simulink model "EMPlanner_cs_old"  (R2023a)
settings: Solver=ode5  StartTime=0.0  StopTime=60  FixedStep=1/1000  RelTol=1e-3
PreLoadFcn:
  | mbxruntime.callbacks.PreLoadFcn(bdroot);
PostLoadFcn:
  | mbxruntime.callbacks.PostLoadFcn(bdroot);
InitFcn:
  | mbxruntime.callbacks.InitFcn(bdroot);
StartFcn:
  | mbxruntime.callbacks.StartFcn(bdroot);
StopFcn:
  | mbxruntime.callbacks.StopFcn(bdroot);
model workspace: external: MAT-File .\EMPlanner_cs_hws.mat (data not in the file)
values from neighbouring files (symbols this model uses):
  c_factor = 43.75    [emplanner_init.m]
  cf = -64276.3    [emplanner_init.m]
  cr = -64276.3    [emplanner_init.m]
  KD_PID_distance = 0.0    (= 0)    [emplanner_init.m]
  KD_PID_speed = 0    [emplanner_init.m]
  KI_PID_distance = 0.0    (= 0)    [emplanner_init.m]
  KI_PID_speed = 0    [emplanner_init.m]
  KP_PID_distance = 0.5    [emplanner_init.m]
  KP_PID_speed = 1.8    [emplanner_init.m]
  la = 0.5989    [emplanner_init.m]
  lb = 1.1979-0.5989    (= 0.599)    [emplanner_init.m]
  LQR_K1 = k(:,1)'    [emplanner_init.m]
  LQR_K2 = k(:,2)'    [emplanner_init.m]
  LQR_K3 = k(:,3)'    [emplanner_init.m]
  LQR_K4 = k(:,4)'    [emplanner_init.m]
  m = 375.8    [emplanner_init.m]
  vx_break_point = zeros(1,5000)    [emplanner_init.m]
undefined symbols (not defined in the file or in its folder): aubr, DiscIntNeverNeededParam, EMPlanner_cs_27357ced727cddc2, EMPlanner_cs_3a309230b46bf2dd, EMPlanner_cs_4725e6271df7126f, EMPlanner_cs_7cd0898d5750b5ce, EMPlanner_cs_9531ed1ae61b92f2, EMPlanner_cs_Box_10_Dynamics_Empty_STATE_Box_10_Pitch0, EMPlanner_cs_Box_10_Dynamics_Empty_STATE_Box_10_Roll0, EMPlanner_cs_Box_10_Dynamics_Empty_STATE_Box_10_x0, EMPlanner_cs_Box_10_Dynamics_Empty_STATE_Box_10_y0, EMPlanner_cs_Box_10_Dynamics_Empty_STATE_Box_10_Yaw0, EMPlanner_cs_Box_10_Dynamics_Empty_STATE_Box_10_z0, EMPlanner_cs_Box_1_Path_pathUniqueID, EMPlanner_cs_Box_1_SpeedProfile_speedProfileUniqueID, EMPlanner_cs_Box_2_Path_pathUniqueID, EMPlanner_cs_Box_2_SpeedProfile_speedProfileUniqueID, EMPlanner_cs_Box_3_Path_pathUniqueID, EMPlanner_cs_Box_3_SpeedProfile_speedProfileUniqueID, EMPlanner_cs_Box_4_Path_pathUniqueID, EMPlanner_cs_Box_4_SpeedProfile_speedProfileUniqueID, EMPlanner_cs_Box_5_Dynamics_Empty_STATE_Box_5_Pitch0, EMPlanner_cs_Box_5_Dynamics_Empty_STATE_Box_5_Roll0, EMPlanner_cs_Box_5_Dynamics_Empty_STATE_Box_5_x0, EMPlanner_cs_Box_5_Dynamics_Empty_STATE_Box_5_y0, EMPlanner_cs_Box_5_Dynamics_Empty_STATE_Box_5_Yaw0, EMPlanner_cs_Box_5_Dynamics_Empty_STATE_Box_5_z0, EMPlanner_cs_Box_6_Path_pathUniqueID, EMPlanner_cs_Box_6_SpeedProfile_speedProfileUniqueID, EMPlanner_cs_Box_7_Dynamics_Empty_STATE_Box_7_Pitch0, EMPlanner_cs_Box_7_Dynamics_Empty_STATE_Box_7_Roll0, EMPlanner_cs_Box_7_Dynamics_Empty_STATE_Box_7_x0, EMPlanner_cs_Box_7_Dynamics_Empty_STATE_Box_7_y0, EMPlanner_cs_Box_7_Dynamics_Empty_STATE_Box_7_Yaw0, EMPlanner_cs_Box_7_Dynamics_Empty_STATE_Box_7_z0, EMPlanner_cs_Box_8_Dynamics_Empty_STATE_Box_8_Pitch0, EMPlanner_cs_Box_8_Dynamics_Empty_STATE_Box_8_Roll0, EMPlanner_cs_Box_8_Dynamics_Empty_STATE_Box_8_x0, EMPlanner_cs_Box_8_Dynamics_Empty_STATE_Box_8_y0, EMPlanner_cs_Box_8_Dynamics_Empty_STATE_Box_8_Yaw0, EMPlanner_cs_Box_8_Dynamics_Empty_STATE_Box_8_z0, EMPlanner_cs_Box_9_Dynamics_Empty_STATE_Box_9_Pitch0, EMPlanner_cs_Box_9_Dynamics_Empty_STATE_Box_9_Roll0, EMPlanner_cs_Box_9_Dynamics_Empty_STATE_Box_9_x0, EMPlanner_cs_Box_9_Dynamics_Empty_STATE_Box_9_y0, EMPlanner_cs_Box_9_Dynamics_Empty_STATE_Box_9_Yaw0, EMPlanner_cs_Box_9_Dynamics_Empty_STATE_Box_9_z0, EMPlanner_cs_dca7ae789a013f83, global_path_x, global_path_y, mbxruntime, rack_displacement, right_wheel_ground, tablebr, vubr
libraries: PreScanSimulinkLibrary x12, Solver_SF x1
(part 5 of 9)

== system EMPlanner_cs_old/modular_bus_1/Dynamics_UserSpecified/MuxState ==
  note: mode: Dynamics
  note: mode: Positioning
  note: mode: Dynamics
      | VelVEHICLE
      | wrt VEH
  note: AnglesVEHICLE
      | wrtGLOB
  note: For state mode 'Dynamic' positions
      | are not taken into account, as they
      | are computed by integrating velocity.
      | Click annotation for Help.
  x [m] : Inport  SampleTime=TimeStep
  y [m] : Inport  Port=2  SampleTime=TimeStep
  z [m] : Inport  Port=3  SampleTime=TimeStep
  dx [m/s] : Inport  Port=4  SampleTime=TimeStep
  dy [m/s] : Inport  Port=5  SampleTime=TimeStep
  dz [m/s] : Inport  Port=6  SampleTime=TimeStep
  R [rad] : Inport  Port=7  SampleTime=TimeStep
  P [rad] : Inport  Port=8  SampleTime=TimeStep
  Y [rad] : Inport  Port=9  SampleTime=TimeStep
  Constant : Constant  DisableCoverage=on  Value=positioningmode
  Discrete-Time Integrator : DiscreteIntegrator  SampleTime=TimeStep  ICPrevOutput=DiscIntNeverNeededParam  ICPrevScaledInput=DiscIntNeverNeededParam
  Ground : Ground
  Ground1 : Ground
  Mux1 : Mux  Inputs=[3 3]
  Mux2 : Mux  Inputs=3
  Mux3 : Mux  Inputs=3
  Mux4 : Mux  Inputs=3
  Mux5 : Mux  Inputs=[3 3]
  Mux6 : Mux  Inputs=[6 3]
  Switch : Switch  Threshold=0.5  SaturateOnIntegerOverflow=off  InputSameDT=off
  Transformation_BODY2GLOBAL : PreScanSimulinkLibrary/Simple_Vehicle_Dynamics/Chassis/MuxDynState/Transformation_BODY2GLOBAL  SystemSampleTime=-1  VariantActivationTime=update diagram  Latency=0  AutoFrameSizeCalculation=off
  mux3 : Mux  Inputs=3
  state : Outport
  wires:
  Constant/1 -> Switch/2
  Mux6/1 -> state/1
  Mux4/1 -> Mux1/1
  Mux5/1 -> Switch/3
  Mux1/1 -> Switch/1
  Switch/1 -> Mux6/1  "PosVeh wrt  GLOB"
  P [rad]/1 -> Mux3/2
  R [rad]/1 -> Mux3/1
  dz [m/s]/1 -> Mux2/3
  dy [m/s]/1 -> Mux2/2
  dx [m/s]/1 -> Mux2/1
  z [m]/1 -> Mux4/3
  y [m]/1 -> Mux4/2
  x [m]/1 -> Mux4/1
  Ground1/1 -> mux3/2  "pitch"
  Y [rad]/1 -> mux3/3, Mux3/3  "yaw"
  Mux3/1 -> Mux6/2
  Transformation_BODY2GLOBAL/1 -> Discrete-Time Integrator/1, Mux5/2  "VelVEH wrt  GLOB"
  mux3/1 -> Transformation_BODY2GLOBAL/2
  Ground/1 -> mux3/1  "roll"
  Mux2/1 -> Mux1/2, Transformation_BODY2GLOBAL/1
  Discrete-Time Integrator/1 -> Mux5/1  "PosVEH wrt  GLOB"

== system EMPlanner_cs_old/modular_bus_1/Dynamics_UserSpecified/STATE_modular_bus_1 ==
  State : Inport  SampleTime=TimeStep
  Bus Creator : BusCreator  Inputs=15  OutDataTypeStr=Bus: PRESCAN_STATEACTUATORDATA  NonVirtualBus=on
  Constant : Constant  Value=0
  Demux : Demux  Outputs=15
  Mux : Mux  Inputs=3
  Mux1 : Mux  Inputs=3
  Mux2 : Mux  Inputs=3
  iniBODYAngles wrtVEH [rad] : Constant  Value=Roll0  SampleTime=TimeStep
  iniBODYAngles wrtVEH [rad]1 : Constant  Value=Pitch0  SampleTime=TimeStep
  iniVEHAngles wrtGLOB [rad] : Constant  Value=Yaw0  SampleTime=TimeStep
  iniVEHposition wrtGLOB [m] : Constant  Value=x0  SampleTime=TimeStep
  iniVEHposition wrtGLOB [m]1 : Constant  Value=y0  SampleTime=TimeStep
  iniVEHposition wrtGLOB [m]2 : Constant  Value=z0  SampleTime=TimeStep
  state2FullState : PreScanSimulinkLibrary/state2FullState  SystemSampleTime=-1  VariantActivationTime=update diagram  Latency=0  AutoFrameSizeCalculation=off
  StateBus : Outport  OutDataTypeStr=Bus: PRESCAN_STATEACTUATORDATA
  wires:
  Mux2/1 -> state2FullState/4
  iniVEHAngles wrtGLOB [rad]/1 -> Mux2/3
  Mux1/1 -> state2FullState/3
  Constant/1 -> Mux2/1, Mux2/2, Mux1/3
  iniBODYAngles wrtVEH [rad]1/1 -> Mux1/2
  iniBODYAngles wrtVEH [rad]/1 -> Mux1/1
  Mux/1 -> state2FullState/2
  iniVEHposition wrtGLOB [m]2/1 -> Mux/3
  iniVEHposition wrtGLOB [m]/1 -> Mux/1
  iniVEHposition wrtGLOB [m]1/1 -> Mux/2
  Demux/15 -> Bus Creator/15  "AngularVelocityYaw"
  Demux/14 -> Bus Creator/14  "AngularVelocityPitch"
  Demux/13 -> Bus Creator/13  "AngularVelocityRoll"
  Demux/12 -> Bus Creator/12  "OrientationYaw"
  Demux/11 -> Bus Creator/11  "OrientationPitch"
  Demux/10 -> Bus Creator/10  "OrientationRoll"
  Demux/9 -> Bus Creator/9  "AccelerationZ"
  Demux/8 -> Bus Creator/8  "AccelerationY"
  Demux/7 -> Bus Creator/7  "AccelerationX"
  Demux/6 -> Bus Creator/6  "VelocityZ"
  Demux/5 -> Bus Creator/5  "VelocityY"
  Demux/4 -> Bus Creator/4  "VelocityX"
  Demux/3 -> Bus Creator/3  "PositionZ"
  Demux/2 -> Bus Creator/2  "PositionY"
  Demux/1 -> Bus Creator/1  "PositionX"
  state2FullState/1 -> Demux/1
  State/1 -> state2FullState/1
  Bus Creator/1 -> StateBus/1

== system EMPlanner_cs_old/modular_bus_1/SELF_Demux/compas converter ==
  rotz [rad] : Inport
  cart2compas : Subsystem
  rad2deg : Gain  Gain=180/pi
  heading [deg] : Outport
  wires:
  rad2deg/1 -> cart2compas/1(Angle [deg])
  rotz [rad]/1 -> rad2deg/1
  cart2compas/1(heading [deg]) -> heading [deg]/1

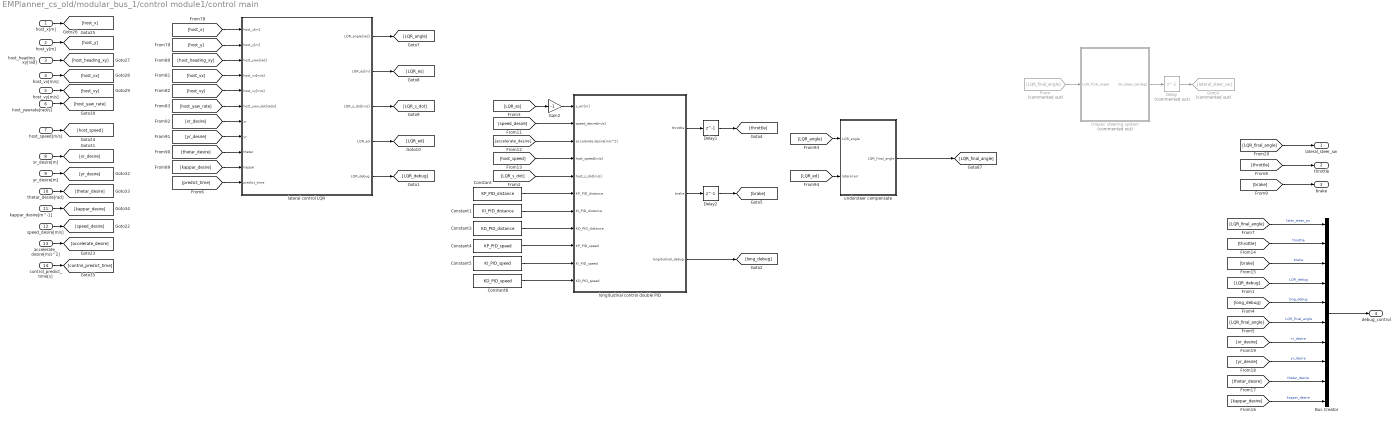
== system EMPlanner_cs_old/modular_bus_1/control module1/control main ==
  host_x[m] : Inport
  host_y[m] : Inport  Port=2
  host_heading_xy[rad] : Inport  Port=3
  host_vx[m/s] : Inport  Port=4
  host_vy[m/s] : Inport  Port=5
  host_yawrate[rad/s] : Inport  Port=6
  host_speed[m/s] : Inport  Port=7
  xr_desire[m] : Inport  Port=8
  yr_desire[m] : Inport  Port=9
  thetar_desire[rad] : Inport  Port=10
  kappar_desire[m^-1] : Inport  Port=11
  speed_desire[m/s] : Inport  Port=12
  accelerate_desire[m/s^2] : Inport  Port=13
  control_predict_time[s] : Inport  Port=14
  Bus Creator : BusCreator  Inputs=10
  Constant : Constant  Value=KP_PID_distance
  Constant1 : Constant  Value=KI_PID_distance
  Constant3 : Constant  Value=KD_PID_distance
  Constant4 : Constant  Value=KP_PID_speed
  Constant5 : Constant  Value=KI_PID_speed
  Constant6 : Constant  Value=KD_PID_speed
  Delay : Delay  Commented=on  DelayLength=1
  Delay1 : Delay  DelayLength=1
  Delay2 : Delay  DelayLength=1
  From : From  Commented=on  GotoTag=LQR_final_angle
  Gain2 : Gain  Gain=-1
  Goto3 : Goto  Commented=on  GotoTag=lateral_steer_sw
  chassic steering system : Subsystem  Commented=on
  lateral control LQR : Subsystem
  longitudinal control double PID : Subsystem
  understeer compensate : Subsystem
  lateral_steer_sw : Outport
  throttle : Outport  Port=2
  brake : Outport  Port=3
  debug_control : Outport  Port=4
  wires:
  [kappar_desire] -> Bus Creator/10  "kappar_desire"
  [thetar_desire] -> Bus Creator/9  "thetar_desire"
  [yr_desire] -> Bus Creator/8  "yr_desire"
  [xr_desire] -> Bus Creator/7  "xr_desire"
  Bus Creator/1 -> debug_control/1
  [LQR_final_angle] -> Bus Creator/6  "LQR_final_angle"
  [long_debug] -> Bus Creator/5  "long_debug"
  [LQR_debug] -> Bus Creator/4  "LQR_debug"
  [brake] -> Bus Creator/3  "brake"
  [throttle] -> Bus Creator/2  "throttle"
  [LQR_final_angle] -> Bus Creator/1  "later_steer_sw"
  [brake] -> brake/1
  [throttle] -> throttle/1
  [LQR_final_angle] -> lateral_steer_sw/1
  Delay2/1 -> [brake]
  Delay1/1 -> [throttle]
  Delay/1 -> Goto3/1
  longitudinal control double PID/3(longitudinal_debug) -> [long_debug]
  lateral control LQR/5(LQR_debug) -> [LQR_debug]
  longitudinal control double PID/2(brake) -> Delay2/1
  longitudinal control double PID/1(throttle) -> Delay1/1
  chassic steering system/1(lat_steer_sw[deg]) -> Delay/1
  From/1 -> chassic steering system/1(LQR_final_angle)
  [LQR_es] -> Gain2/1
  Gain2/1 -> longitudinal control double PID/1(s_err[m])
  Constant6/1 -> longitudinal control double PID/11(KD_PID_speed)
  speed_desire[m/s]/1 -> [speed_desire]
  control_predict_time[s]/1 -> [control_predict_time]
  host_speed[m/s]/1 -> [host_speed]
  host_vy[m/s]/1 -> [host_vy]
  host_y[m]/1 -> [host_y]
  [host_yaw_rate] -> lateral control LQR/6(host_yaw_dot[rad/s])
  yr_desire[m]/1 -> [yr_desire]
  kappar_desire[m^-1]/1 -> [kappar_desire]
  host_yawrate[rad/s]/1 -> [host_yaw_rate]
  [kappar_desire] -> lateral control LQR/10(kappar)
  [host_heading_xy] -> lateral control LQR/3(host_yaw[rad])
  [thetar_desire] -> lateral control LQR/9(thetar)
  lateral control LQR/4(LQR_ed) -> [LQR_ed]
  [speed_desire] -> longitudinal control double PID/2(speed_desire[m/s])
  host_vx[m/s]/1 -> [host_vx]
  [predict_time] -> lateral control LQR/11(predict_time)
  [host_speed] -> longitudinal control double PID/4(host_speed[m/s])
  Constant4/1 -> longitudinal control double PID/9(KP_PID_speed)
  Constant5/1 -> longitudinal control double PID/10(KI_PID_speed)
  Constant3/1 -> longitudinal control double PID/8(KD_PID_distance)
  Constant/1 -> longitudinal control double PID/6(KP_PID_distance)
  lateral control LQR/3(LQR_s_dot[m/s]) -> [LQR_s_dot]
  [LQR_ed] -> understeer compensate/2(lateral err)
  host_heading_xy[rad]/1 -> [host_heading_xy]
  lateral control LQR/2(LQR_es[m]) -> [LQR_es]
  [host_vy] -> lateral control LQR/5(host_vy[m/s])
  xr_desire[m]/1 -> [xr_desire]
  [LQR_angle] -> understeer compensate/1(LQR_angle)
  [yr_desire] -> lateral control LQR/8(yr)
  [LQR_s_dot] -> longitudinal control double PID/5(host_s_dot[m/s])
  [host_y] -> lateral control LQR/2(host_y[m])
  accelerate_desire[m/s^2]/1 -> [accelerate_desire]
  [xr_desire] -> lateral control LQR/7(xr)
  [host_x] -> lateral control LQR/1(host_x[m])
  [accelerate_desire] -> longitudinal control double PID/3(accelerate desire[m/s^2])
  Constant1/1 -> longitudinal control double PID/7(KI_PID_distance)
  thetar_desire[rad]/1 -> [thetar_desire]
  [host_vx] -> lateral control LQR/4(host_vx[m/s])
  lateral control LQR/1(LQR_angle[rad]) -> [LQR_angle]
  host_x[m]/1 -> [host_x]
  understeer compensate/1(LQR_final_angle) -> [LQR_final_angle]

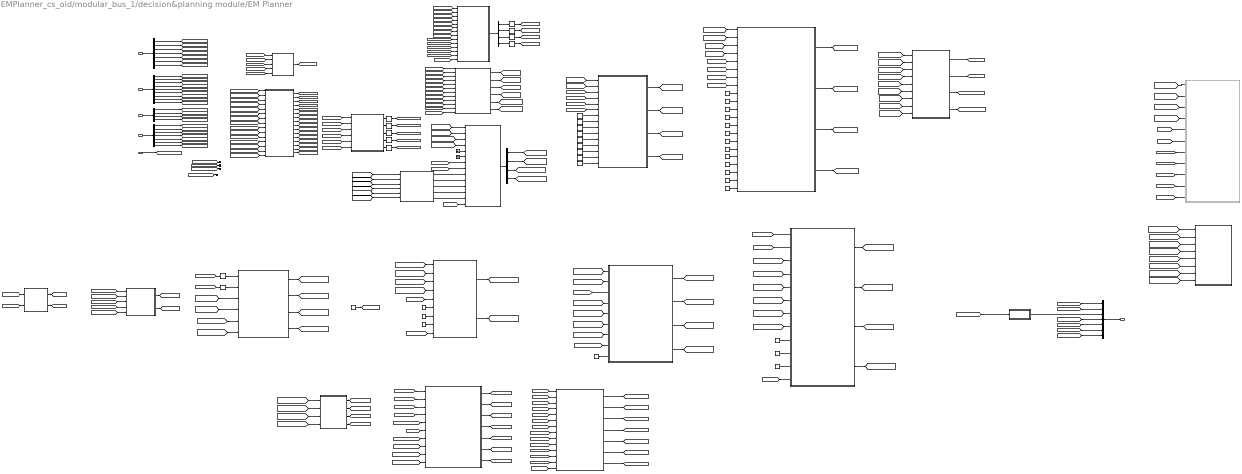
== system EMPlanner_cs_old/modular_bus_1/decision&planning module/EM Planner ==
  referenceline info : Inport
  location info : Inport  Port=2
  perception info : Inport  Port=3
  pre_planning info : Inport  Port=4
  current time : Inport  Port=5
  Bus Creator : BusCreator  Inputs=7
  Bus Selector : BusSelector  OutputSignals=referenceline_x,referenceline_y,referenceline_heading,referenceline_kappa,origin_match_point_index,origin_x,origin_y
  Bus Selector1 : BusSelector  OutputSignals=host_x,host_y,host_heading_xy,host_vx,host_vy,host_yawrate,host_speed,host_ax,host_ay
  Bus Selector2 : BusSelector  OutputSignals=obs_x_set_gcs,obs_y_set_gcs,obs_velocity_set_gcs,obs_heading_set_gcs
  Bus Selector3 : BusSelector  OutputSignals=trajectory_x_gcs,trajectory_y_gcs,trajectory_heading_gcs,trajectory_kappa_gcs,trajectory_speed_gcs,trajectory_accel_gcs,trajectory_time_gcs
  Bus Selector4 : BusSelector  OutputSignals=s_set,l_set,dl_set,ddl_set
  Bus Selector5 : BusSelector  OutputSignals=s_set,l_set,s_dot_set,l_dot_set
  Cartesian2Frenet : Subsystem
  Cartesian2Frenet1 : Subsystem
  Constant : Constant  Value=1e6
  Constant1 : Constant  Value=2000
  Constant10 : Constant  Value=0.1
  Constant11 : Constant  Value=0.02
  Constant12 : Constant  Value=2
  Constant13 : Constant  Value=25000
  Constant14 : Constant  Value=50
  Constant15 : Constant  Value=20
  Constant{7,16..19} (5 alike) : Constant  Value=15
  Constant2 : Constant  Value=2
  Constant20 : Constant  Value=3
  Constant21 : Constant  Value=3
  Constant22 : Constant  Value=1.63
  Constant23 : Constant  Value=5
  Constant24 : Constant  Value=4000
  Constant25 : Constant  Value=100
  Constant26 : Constant  Value=10000000
  Constant27 : Constant  Value=0.2*9.8
  Constant28 : Constant  Value=50
  Constant29 : Constant  Value=500
  Constant3 : Constant  Value=3
  Constant4 : Constant  Value=10
  Constant5 : Constant  Value=11
  Constant6 : Constant  Value=4
  Constant8 : Constant
  Constant9 : Constant  Value=10
  Delay : Delay  DelayLength=1
  Delay1 : Delay  DelayLength=1
  Frenet2Cartesian task : MATLAB Function  TreatAsAtomicUnit=on
  Ground : Ground
  Ground1 : Ground
  MATLAB Function : MATLAB Function  TreatAsAtomicUnit=on
  MATLAB Function1 : MATLAB Function  TreatAsAtomicUnit=on
  MATLAB Function2 : MATLAB Function  TreatAsAtomicUnit=on
  MATLAB Function5 : MATLAB Function  TreatAsAtomicUnit=on
  Selector{1..9} (9 alike) : Selector  InputPortWidth=128  IndexOptions=Index vector (dialog)  Indices=1  OutputSizes=1
  Terminator_{1..4} (4 alike) : Terminator
  calc path length and map between point and s : MATLAB Function  TreatAsAtomicUnit=on
  calc plan start info and stitch trajectory : MATLAB Function  TreatAsAtomicUnit=on
  calc speed planning start condition : MATLAB Function  TreatAsAtomicUnit=on
  generate convex space : MATLAB Function  TreatAsAtomicUnit=on
  generate st graph : MATLAB Function  TreatAsAtomicUnit=on
  genrate index to s : MATLAB Function  TreatAsAtomicUnit=on
  increase st point count : MATLAB Function  TreatAsAtomicUnit=on
  obs : Subsystem
  path and speed merge : MATLAB Function  TreatAsAtomicUnit=on
  path decision task : Subsystem
  path planning task : Subsystem
  plot : MATLAB Function  Commented=on  TreatAsAtomicUnit=on
  spee planning with quadratic programming (qp) : MATLAB Function  TreatAsAtomicUnit=on
  speed decision with dynamic planning(dp) : MATLAB Function  TreatAsAtomicUnit=on
  stitch trajectory : MATLAB Function  TreatAsAtomicUnit=on
  EM Planner result : Outport
  wires:
  [pre_trajectory_time] -> Terminator_4/1
  [pre_trajectory_speed_gcs] -> Terminator_3/1
  [pre_trajectory_y_gcs] -> Terminator_2/1
  [pre_trajectory_x_gcs] -> Terminator_1/1
  [reference_speed] -> spee planning with quadratic programming (qp)/12(speed_reference)
  [reference_speed] -> speed decision with dynamic planning(dp)/5(reference_speed_unlimit)
  Constant23/1 -> [reference_speed]
  [relative_time_init] -> MATLAB Function5/4(qp_speed_t)
  [qp_s_init] -> MATLAB Function5/3(qp_speed_s)
  [dp_speed_s] -> MATLAB Function5/1(dp_speed_s)
  [dp_speed_t] -> MATLAB Function5/2(dp_speed_t)
  [plan_start_s_dot2] -> spee planning with quadratic programming (qp)/2(plan_start_s_dot2)
  Constant29/1 -> spee planning with quadratic programming (qp)/11(w_cost_jerk)
  Constant28/1 -> spee planning with quadratic programming (qp)/10(w_cost_v_ref)
  Constant9/1 -> spee planning with quadratic programming (qp)/9(w_cost_s_dot2)
  [relative_time_init] -> increase st point count/4(relative_time_init)
  [qp_s_dot_init] -> increase st point count/2(s_dot_init)
  [qp_s_dot2_init] -> increase st point count/3(s_dot2_init)
  [qp_s_init] -> increase st point count/1(s_init)
  spee planning with quadratic programming (qp)/4(relative_time_init) -> [relative_time_init]
  spee planning with quadratic programming (qp)/3(qp_s_dot2_init) -> [qp_s_dot2_init]
  spee planning with quadratic programming (qp)/2(qp_s_dot_init) -> [qp_s_dot_init]
  spee planning with quadratic programming (qp)/1(qp_s_init) -> [qp_s_init]
  [s_dot_ub] -> spee planning with quadratic programming (qp)/8(s_dot_ub)
  [s_dot_lb] -> spee planning with quadratic programming (qp)/7(s_dot_lb)
  [s_ub] -> spee planning with quadratic programming (qp)/6(s_ub)
  [s_lb] -> spee planning with quadratic programming (qp)/5(s_lb)
  [dp_speed_t] -> spee planning with quadratic programming (qp)/4(dp_speed_t)
  [dp_speed_s] -> spee planning with quadratic programming (qp)/3(dp_speed_s)
  [plan_start_s_dot] -> spee planning with quadratic programming (qp)/1(plan_start_s_dot)
  [obs_st_t_out_set] -> MATLAB Function5/8(obs_t_out_set)
  [obs_st_t_in_set] -> MATLAB Function5/7(obs_t_in_set)
  [obs_st_s_out_set] -> MATLAB Function5/6(obs_s_out_set)
  [obs_st_s_in_set] -> MATLAB Function5/5(obs_s_in_set)
  speed decision with dynamic planning(dp)/1(dp_speed_s) -> [dp_speed_s]
  generate convex space/4(s_dot_ub) -> [s_dot_ub]
  generate convex space/3(s_dot_lb) -> [s_dot_lb]
  generate convex space/2(s_ub) -> [s_ub]
  generate convex space/1(s_lb) -> [s_lb]
  Constant27/1 -> generate convex space/9(max_lateral_accel)
  [trajectory_kappa_init] -> generate convex space/8(trajectory_kappa_init)
  [obs_st_s_out_set] -> generate convex space/5(obs_st_s_out_set)
  [obs_st_t_in_set] -> generate convex space/6(obs_st_t_in_set)
  [obs_st_t_out_set] -> generate convex space/7(obs_st_t_out_set)
  [obs_st_s_in_set] -> generate convex space/4(obs_st_s_in_set)
  [dp_speed_t] -> generate convex space/2(dp_speed_t)
  [dp_speed_s] -> generate convex space/1(dp_speed_s)
  speed decision with dynamic planning(dp)/2(dp_speed_t) -> [dp_speed_t]
  [path_index2s] -> generate convex space/3(path_index2s)
  [plan_start_s_dot] -> speed decision with dynamic planning(dp)/9(plan_start_s_dot)
  Constant26/1 -> speed decision with dynamic planning(dp)/8(w_cost_obs)
  Constant25/1 -> speed decision with dynamic planning(dp)/7(w_cost_accel)
  Constant24/1 -> speed decision with dynamic planning(dp)/6(w_cost_ref_speed)
  [obs_st_t_out_set] -> speed decision with dynamic planning(dp)/4(obs_st_t_out_set)
  [obs_st_t_in_set] -> speed decision with dynamic planning(dp)/3(obs_st_t_in_set)
  [obs_st_s_out_set] -> speed decision with dynamic planning(dp)/2(obs_st_s_out_set)
  [obs_st_s_in_set] -> speed decision with dynamic planning(dp)/1(obs_st_s_in_set)
  generate st graph/2(obs_st_s_out_set) -> [obs_st_s_out_set]
  generate st graph/4(obs_st_t_out_set) -> [obs_st_t_out_set]
  generate st graph/3(obs_st_t_in_set) -> [obs_st_t_in_set]
  generate st graph/1(obs_st_s_in_set) -> [obs_st_s_in_set]
  [dynamic_obs_l_dot_set] -> generate st graph/6(dynamic_obs_l_dot_set)
  [dynamic_obs_s_dot_set] -> generate st graph/5(dynamic_obs_s_dot_set)
  [dynamic_obs_l_set] -> generate st graph/4(dynamic_obs_l_set)
  [dynamic_obs_s_set] -> generate st graph/3(dynamic_obs_s_set)
  stitch trajectory/7(trajectory_time_final) -> [trajectory_time_final]
  Delay1/1 -> generate st graph/2(pre_trajectory_t)
  Delay/1 -> generate st graph/1(pre_trajectory_s)
  [relative_time] -> Delay1/1
  [s] -> Delay/1
  [path_index2s] -> Cartesian2Frenet1/14(index2s)
  Bus Selector5/4 -> [dynamic_obs_l_dot_set]  "<l_dot_set>"
  Bus Selector5/3 -> [dynamic_obs_s_dot_set]  "<s_dot_set>"
  Bus Selector5/2 -> [dynamic_obs_l_set]  "<l_set>"
  Bus Selector5/1 -> [dynamic_obs_s_set]  "<s_set>"
  Cartesian2Frenet1/1(Cartesian2FrenetOut) -> Bus Selector5/1
  [dynamic_obs_x_set] -> MATLAB Function1/1(x_set)
  [dynamic_obs_y_set] -> MATLAB Function1/2(y_set)
  [trajectory_kappa_init] -> MATLAB Function1/6(frenet_path_kappa)
  [trajectory_heading_init] -> MATLAB Function1/5(frenet_path_heading)
  [trajectory_y_init] -> MATLAB Function1/4(frenet_path_y)
  [trajectory_x_init] -> MATLAB Function1/3(frenet_path_x)
  MATLAB Function1/5(proj_kappa_set) -> Cartesian2Frenet1/13(proj_kappa_set)
  MATLAB Function1/4(proj_heading_set) -> Cartesian2Frenet1/12(proj_heading_set)
  MATLAB Function1/3(proj_y_set) -> Cartesian2Frenet1/11(proj_y_set)
  MATLAB Function1/2(proj_x_set) -> Cartesian2Frenet1/10(proj_x_set)
  MATLAB Function1/1(match_point_index_set) -> Cartesian2Frenet1/9(proj_match_point_index_set)
  [trajectory_y_init] -> Cartesian2Frenet1/8(frenet_path_y)
  [trajectory_x_init] -> Cartesian2Frenet1/7(frenet_path_x)
  Ground1/1 -> Cartesian2Frenet1/6(ay_set)
  Ground/1 -> Cartesian2Frenet1/5(ax_set)
  [dynamic_obs_x_set] -> Cartesian2Frenet1/1(x_set)
  [dynamic_obs_y_set] -> Cartesian2Frenet1/2(y_set)
  [dynamic_obs_vx_set] -> Cartesian2Frenet1/3(vx_set)
  [dynamic_obs_vy_set] -> Cartesian2Frenet1/4(vy_set)
  [relative_time] -> path and speed merge/4(relative_time)
  [s_dot2] -> path and speed merge/3(s_dot2)
  [s] -> path and speed merge/1(s)
  [s_dot] -> path and speed merge/2(s_dot)
  increase st point count/4(relative_time) -> [relative_time]
  increase st point count/1(s) -> [s]
  increase st point count/2(s_dot) -> [s_dot]
  increase st point count/3(s_dot2) -> [s_dot2]
  obs/6(dynamic_obs_vy_set) -> [dynamic_obs_vy_set]
  obs/5(dynamic_obs_vx_set) -> [dynamic_obs_vx_set]
  obs/4(dynamic_obs_y_set) -> [dynamic_obs_y_set]
  obs/3(dynamic_obs_x_set) -> [dynamic_obs_x_set]
  MATLAB Function/1(y) -> Bus Creator/3  "trajectory_heading_gcs"
  [plan_start_s] -> path planning task/5(plan_start_s)
  [qp_path_l_final] -> plot/4(qp_l)
  [qp_path_s_final] -> plot/3(qp_s)
  [qp_path_s_final] -> Frenet2Cartesian task/1(s_set)
  [qp_path_dl_final] -> Frenet2Cartesian task/3(dl_set)
  [qp_path_l_final] -> Frenet2Cartesian task/2(l_set)
  [qp_path_ddl_final] -> Frenet2Cartesian task/4(ddl_set)
  path planning task/4(qp_path_ddl_final) -> [qp_path_ddl_final]
  path planning task/3(qp_path_dl_final) -> [qp_path_dl_final]
  path planning task/2(qp_path_l_final) -> [qp_path_l_final]
  path planning task/1(qp_path_s_final) -> [qp_path_s_final]
  Constant11/1 -> path planning task/21(delta_ddl_max)
  Constant10/1 -> path planning task/20(delta_dl_max)
  [static_obs_l_set] -> path planning task/4(static_obs_l_set)
  [static_obs_s_set] -> path planning task/3(static_obs_s_set)
  Constant2/1 -> path decision task/9(dp_cost_ddl)
  Constant1/1 -> path decision task/8(dp_cost_dl)
  Constant/1 -> path decision task/7(dp_cost_collision)
  Constant3/1 -> path decision task/10(dp_cost_dddl)
  Constant4/1 -> path decision task/11(dp_cost_ref)
  Constant5/1 -> path decision task/12(dp_row)
  Constant6/1 -> path decision task/13(dp_col)
  Constant7/1 -> path decision task/14(dp_sample_s)
  Constant8/1 -> path decision task/15(dp_sample_l)
  Constant12/1 -> path planning task/9(qp_cost_l)
  Constant13/1 -> path planning task/10(qp_cost_dl)
  Constant14/1 -> path planning task/11(qp_cost_ddl)
  Constant15/1 -> path planning task/12(qp_cost_dddl)
  Constant16/1 -> path planning task/13(qp_cost_centre)
  Constant17/1 -> path planning task/14(qp_cost_endl)
  Constant18/1 -> path planning task/15(qp_cost_end_dl)
  Constant19/1 -> path planning task/16(qp_cost_end_ddl)
  Constant20/1 -> path planning task/17(host_d1)
  Constant21/1 -> path planning task/18(host_d2)
  Constant22/1 -> path planning task/19(host_w)
  [plan_start_dl] -> path planning task/7(plan_start_dl)
  [plan_start_ddl] -> path planning task/8(plan_start_ddl)
  [plan_start_l] -> path planning task/6(plan_start_l)
  [dp_path_l_final] -> path planning task/2(dp_path_l_final)
  [dp_path_s_final] -> path planning task/1(dp_path_s_final)
  [plan_start_s] -> path decision task/3(plan_start_s)
  [plan_start_l] -> path decision task/4(plan_start_l)
  [plan_start_dl] -> path decision task/5(plan_start_dl)
  [plan_start_ddl] -> path decision task/6(plan_start_ddl)
  [static_obs_l_set] -> path decision task/2(static_obs_l_set)
  [static_obs_s_set] -> path decision task/1(static_obs_s_set)
  path decision task/4(dp_path_ddl_final) -> [dp_path_ddl_final]
  path decision task/3(dp_path_dl_final) -> [dp_path_dl_final]
  path decision task/2(dp_path_l_final) -> [dp_path_l_final]
  path decision task/1(dp_path_s_final) -> [dp_path_s_final]
  [static_obs_l_set] -> plot/8(obs_l_set)
  [static_obs_s_set] -> plot/7(obs_s_set)
  [plan_start_s] -> plot/9(start_s)
  [plan_start_l] -> plot/10(start_l)
  [plan_start_dl] -> plot/11(start_dl)
  [l_max] -> plot/6(l_max)
  [l_min] -> plot/5(l_min)
  [dp_path_l_final] -> plot/2(dp_l)
  [dp_path_s_final] -> plot/1(dp_s)
  Frenet2Cartesian task/4(kappa_set) -> [trajectory_kappa_init]
  Frenet2Cartesian task/3(heading_set) -> [trajectory_heading_init]
  Frenet2Cartesian task/2(y_set) -> [trajectory_y_init]
  Frenet2Cartesian task/1(x_set) -> [trajectory_x_init]
  [referenceline_kappa] -> Frenet2Cartesian task/8(frenet_path_kappa)
  [referenceline_heading] -> Frenet2Cartesian task/7(frenet_path_heading)
  [referenceline_y] -> Frenet2Cartesian task/6(frenet_path_y)
  [referenceline_x] -> Frenet2Cartesian task/5(frenet_path_x)
  [index2s] -> Frenet2Cartesian task/9(index2s)
  [trajectory_x_init] -> calc path length and map between point and s/1(trajectory_x)
  [trajectory_heading] -> stitch trajectory/3(trajectory_heading)
  [trajectory_time] -> stitch trajectory/7(trajectory_time)
  [trajectory_y_init] -> path and speed merge/8(trajectory_y_init)
  path and speed merge/5(trajectory_speed) -> [trajectory_speed]
  [plan_start_time] -> path and speed merge/5(current_time)
  [trajectory_heading_init] -> path and speed merge/9(trajectory_heading_init)
  path and speed merge/2(trajectory_y) -> [trajectory_y]
  [path_index2s] -> path and speed merge/6(path_s)
  [stitch_kappa_gcs] -> stitch trajectory/11(stitch_kappa)
  path and speed merge/6(trajectory_accel) -> [trajectory_accel]
  [trajectory_y_init] -> calc path length and map between point and s/2(trajectory_y)
  [trajectory_x] -> stitch trajectory/1(trajectory_x)
  [stitch_accel_gcs] -> stitch trajectory/13(stitch_accel)
  [trajectory_kappa_init] -> path and speed merge/10(trajectory_kappa_init)
  calc speed planning start condition/2(plan_start_s_dot2) -> [plan_start_s_dot2]
  calc path length and map between point and s/1(path_s_end) -> [path_s_end]
  [trajectory_y] -> stitch trajectory/2(trajectory_y)
  [trajectory_y_final] -> Bus Creator/2  "trajectory_y_gcs"
  stitch trajectory/5(trajectory_speed_final) -> [trajectory_speed_final]
  path and speed merge/3(trajectory_heading) -> [trajectory_heading]
  [trajectory_kappa_final] -> Bus Creator/4  "trajectory_kappa_gcs"
  stitch trajectory/3(trajectory_heading_final) -> [trajectory_heading_final]
  stitch trajectory/2(trajectory_y_final) -> [trajectory_y_final]
  [trajectory_x_init] -> path and speed merge/7(trajectory_x_init)
  [trajectory_kappa] -> stitch trajectory/4(trajectory_kappa)
  [trajectory_accel] -> stitch trajectory/6(trajectory_accel)
  [trajectory_heading_final] -> MATLAB Function/1(trajectory_heading_final)
  [plan_start_vx_gcs] -> calc speed planning start condition/1(plan_start_vx)
  stitch trajectory/6(trajectory_accel_final) -> [trajectory_accel_final]
  [stitch_y_gcs] -> stitch trajectory/9(stitch_y)
  [trajectory_speed_final] -> Bus Creator/5  "trajectory_speed_gcs"
  [stitch_heading_gcs] -> stitch trajectory/10(stitch_heading)
  [trajectory_accel_final] -> Bus Creator/6  "trajectory_accel_gcs"
  stitch trajectory/1(trajectory_x_final) -> [trajectory_x_final]
  [stitch_x_gcs] -> stitch trajectory/8(stitch_x)
  [trajectory_time_final] -> Bus Creator/7  "trajectory_time_gcs"
  [stitch_speed_gcs] -> stitch trajectory/12(stitch_speed)
  [plan_start_ay_gcs] -> calc speed planning start condition/4(plan_start_ay)
  calc speed planning start condition/1(plan_start_s_dot) -> [plan_start_s_dot]
  [plan_start_ax_gcs] -> calc speed planning start condition/3(plan_start_ax)
  stitch trajectory/4(trajectory_kappa_final) -> [trajectory_kappa_final]
  [trajectory_x_final] -> Bus Creator/1  "trajectory_x_gcs"
  Bus Creator/1 -> EM Planner result/1
  [plan_start_heading_gcs] -> calc speed planning start condition/5(plan_start_heading)
  calc path length and map between point and s/2(path_index2s) -> [path_index2s]
  [stitch_time] -> stitch trajectory/14(stitch_time)
  [plan_start_vy_gcs] -> calc speed planning start condition/2(plan_start_vy)
  path and speed merge/4(trajectory_kappa) -> [trajectory_kappa]
  [trajectory_speed] -> stitch trajectory/5(trajectory_speed)
  path and speed merge/1(trajectory_x) -> [trajectory_x]
  path and speed merge/7(trajectory_time) -> [trajectory_time]
  obs/2(static_obs_l_set) -> [static_obs_l_set]
  obs/1(static_obs_s_set) -> [static_obs_s_set]
  [index2s] -> obs/12(index2s)
  [referenceline_kappa] -> obs/11(referenceline_kappa)
  [referenceline_heading] -> obs/10(referenceline_heading)
  [referenceline_y] -> obs/9(referenceline_y)
  [referenceline_x] -> obs/8(referenceline_x)
  [obs_heading_set_gcs] -> obs/7(obs_heading_set_gcs)
  [obs_velocity_set_gcs] -> obs/6(obs_velocity_set_gcs)
  [obs_y_set_gcs] -> obs/5(obs_y_set_gcs)
  [obs_x_set_gcs] -> obs/4(obs_x_set_gcs)
  [host_heading_xy] -> obs/3(host_heading_xy)
  [host_y] -> obs/2(host_y)
  [host_x] -> obs/1(host_x)
  [index2s] -> Cartesian2Frenet/14(index2s)
  Selector9/1 -> [plan_start_ddl]
  Selector8/1 -> [plan_start_dl]
  Selector7/1 -> [plan_start_l]
  Selector6/1 -> [plan_start_s]
  Bus Selector4/1 -> Selector6/1  "<s_set>"
  Bus Selector4/2 -> Selector7/1  "<l_set>"
  Bus Selector4/3 -> Selector8/1  "<dl_set>"
  Bus Selector4/4 -> Selector9/1  "<ddl_set>"
  Cartesian2Frenet/1(Cartesian2FrenetOut) -> Bus Selector4/1
  [plan_start_proj_kappa] -> Cartesian2Frenet/13(proj_kappa_set)
  [plan_start_proj_heading] -> Cartesian2Frenet/12(proj_heading_set)
  [plan_start_proj_y] -> Cartesian2Frenet/11(proj_y_set)
  [plan_start_proj_x] -> Cartesian2Frenet/10(proj_x_set)
  [plan_start_match_point_index] -> Cartesian2Frenet/9(proj_match_point_index_set)
  [referenceline_y] -> Cartesian2Frenet/8(frenet_path_y)
  [referenceline_x] -> Cartesian2Frenet/7(frenet_path_x)
  [plan_start_ay_gcs] -> Cartesian2Frenet/6(ay_set)
  [plan_start_ax_gcs] -> Cartesian2Frenet/5(ax_set)
  [plan_start_vy_gcs] -> Cartesian2Frenet/4(vy_set)
  [plan_start_vx_gcs] -> Cartesian2Frenet/3(vx_set)
  [plan_start_x_gcs] -> Cartesian2Frenet/1(x_set)
  [plan_start_y_gcs] -> Cartesian2Frenet/2(y_set)
  Selector5/1 -> [plan_start_proj_kappa]
  Selector4/1 -> [plan_start_proj_heading]
  Selector3/1 -> [plan_start_proj_y]
  Selector2/1 -> [plan_start_proj_x]
  Selector1/1 -> [plan_start_match_point_index]
  [referenceline_kappa] -> MATLAB Function2/6(frenet_path_kappa)
  [referenceline_heading] -> MATLAB Function2/5(frenet_path_heading)
  [referenceline_y] -> MATLAB Function2/4(frenet_path_y)
  [referenceline_x] -> MATLAB Function2/3(frenet_path_x)
  [plan_start_y_gcs] -> MATLAB Function2/2(y_set)
  [plan_start_x_gcs] -> MATLAB Function2/1(x_set)
  MATLAB Function2/2(proj_x_set) -> Selector2/1
  MATLAB Function2/4(proj_heading_set) -> Selector4/1
  MATLAB Function2/1(match_point_index_set) -> Selector1/1
  MATLAB Function2/3(proj_y_set) -> Selector3/1
  MATLAB Function2/5(proj_kappa_set) -> Selector5/1
  genrate index to s/1(index2s) -> [index2s]
  [origin_match_point_index] -> genrate index to s/5(origin_match_point_index)
  [origin_y] -> genrate index to s/4(origin_y)
  [origin_x] -> genrate index to s/3(origin_x)
  [referenceline_y] -> genrate index to s/2(path_y)
  [referenceline_x] -> genrate index to s/1(path_x)
  Bus Selector/7 -> [origin_y]  "<origin_y>"
  Bus Selector/6 -> [origin_x]  "<origin_x>"
  Bus Selector/5 -> [origin_match_point_index]  "<origin_match_point_index>"
  calc plan start info and stitch trajectory/16(stitch_time) -> [stitch_time]
  calc plan start info and stitch trajectory/15(stitch_accel) -> [stitch_accel_gcs]
  calc plan start info and stitch trajectory/14(stitch_speed) -> [stitch_speed_gcs]
  calc plan start info and stitch trajectory/13(stitch_kappa) -> [stitch_kappa_gcs]
  calc plan start info and stitch trajectory/12(stitch_heading) -> [stitch_heading_gcs]
  calc plan start info and stitch trajectory/11(stitch_y) -> [stitch_y_gcs]
  calc plan start info and stitch trajectory/10(stitch_x) -> [stitch_x_gcs]
  calc plan start info and stitch trajectory/9(plan_start_time) -> [plan_start_time]
  calc plan start info and stitch trajectory/8(plan_start_ay) -> [plan_start_ay_gcs]
  calc plan start info and stitch trajectory/7(plan_start_ax) -> [plan_start_ax_gcs]
  calc plan start info and stitch trajectory/6(plan_start_vy) -> [plan_start_vy_gcs]
  calc plan start info and stitch trajectory/5(plan_start_vx) -> [plan_start_vx_gcs]
  calc plan start info and stitch trajectory/4(plan_start_kappa) -> [plan_start_kappa_gcs]
  calc plan start info and stitch trajectory/3(plan_start_heading) -> [plan_start_heading_gcs]
  calc plan start info and stitch trajectory/2(plan_start_y) -> [plan_start_y_gcs]
  calc plan start info and stitch trajectory/1(plan_start_x) -> [plan_start_x_gcs]
  [pre_trajectory_heading_gcs] -> calc plan start info and stitch trajectory/3(pre_trajectory_heading)
  [pre_trajectory_kappa_gcs] -> calc plan start info and stitch trajectory/4(pre_trajectory_kappa)
  [pre_trajectory_speed_gcs] -> calc plan start info and stitch trajectory/5(pre_trajectory_velocity)
  [pre_trajectory_accel_gcs] -> calc plan start info and stitch trajectory/6(pre_trajectory_accel)
  [pre_trajectory_time] -> calc plan start info and stitch trajectory/7(pre_trajectory_time)
  [pre_trajectory_y_gcs] -> calc plan start info and stitch trajectory/2(pre_trajectory_y)
  [pre_trajectory_x_gcs] -> calc plan start info and stitch trajectory/1(pre_trajectory_x)
  [current_time] -> calc plan start info and stitch trajectory/8(current_time)
  [host_x] -> calc plan start info and stitch trajectory/9(host_x)
  [host_y] -> calc plan start info and stitch trajectory/10(host_y)
  [host_heading_xy] -> calc plan start info and stitch trajectory/11(host_heading_xy)
  [host_vx_vcs] -> calc plan start info and stitch trajectory/12(host_vx)
  [host_vy_vcs] -> calc plan start info and stitch trajectory/13(host_vy)
  [host_ax_vcs] -> calc plan start info and stitch trajectory/14(host_ax)
  [host_ay_vcs] -> calc plan start info and stitch trajectory/15(host_ay)
  Bus Selector/4 -> [referenceline_kappa]  "<referenceline_kappa>"
  Bus Selector/3 -> [referenceline_heading]  "<referenceline_heading>"
  Bus Selector/2 -> [referenceline_y]  "<referenceline_y>"
  Bus Selector/1 -> [referenceline_x]  "<referenceline_x>"
  Bus Selector1/9 -> [host_ay_vcs]  "<host_ay>"
  Bus Selector1/8 -> [host_ax_vcs]  "<host_ax>"
  Bus Selector1/7 -> [host_speed]  "<host_speed>"
  Bus Selector1/6 -> [host_yawrate]  "<host_yawrate>"
  Bus Selector1/5 -> [host_vy_vcs]  "<host_vy>"
  Bus Selector1/4 -> [host_vx_vcs]  "<host_vx>"
  Bus Selector1/3 -> [host_heading_xy]  "<host_heading_xy>"
  Bus Selector1/2 -> [host_y]  "<host_y>"
  Bus Selector1/1 -> [host_x]  "<host_x>"
  Bus Selector2/4 -> [obs_heading_set_gcs]  "<obs_heading_set_gcs>"
  Bus Selector2/3 -> [obs_velocity_set_gcs]  "<obs_velocity_set_gcs>"
  Bus Selector2/2 -> [obs_y_set_gcs]  "<obs_y_set_gcs>"
  Bus Selector2/1 -> [obs_x_set_gcs]  "<obs_x_set_gcs>"
  Bus Selector3/7 -> [pre_trajectory_time]  "<trajectory_time_gcs>"
  Bus Selector3/6 -> [pre_trajectory_accel_gcs]  "<trajectory_accel_gcs>"
  Bus Selector3/5 -> [pre_trajectory_speed_gcs]  "<trajectory_speed_gcs>"
  Bus Selector3/4 -> [pre_trajectory_kappa_gcs]  "<trajectory_kappa_gcs>"
  Bus Selector3/3 -> [pre_trajectory_heading_gcs]  "<trajectory_heading_gcs>"
  Bus Selector3/2 -> [pre_trajectory_y_gcs]  "<trajectory_y_gcs>"
  Bus Selector3/1 -> [pre_trajectory_x_gcs]  "<trajectory_x_gcs>"
  current time/1 -> [current_time]
  pre_planning info/1 -> Bus Selector3/1
  perception info/1 -> Bus Selector2/1
  location info/1 -> Bus Selector1/1
  referenceline info/1 -> Bus Selector/1

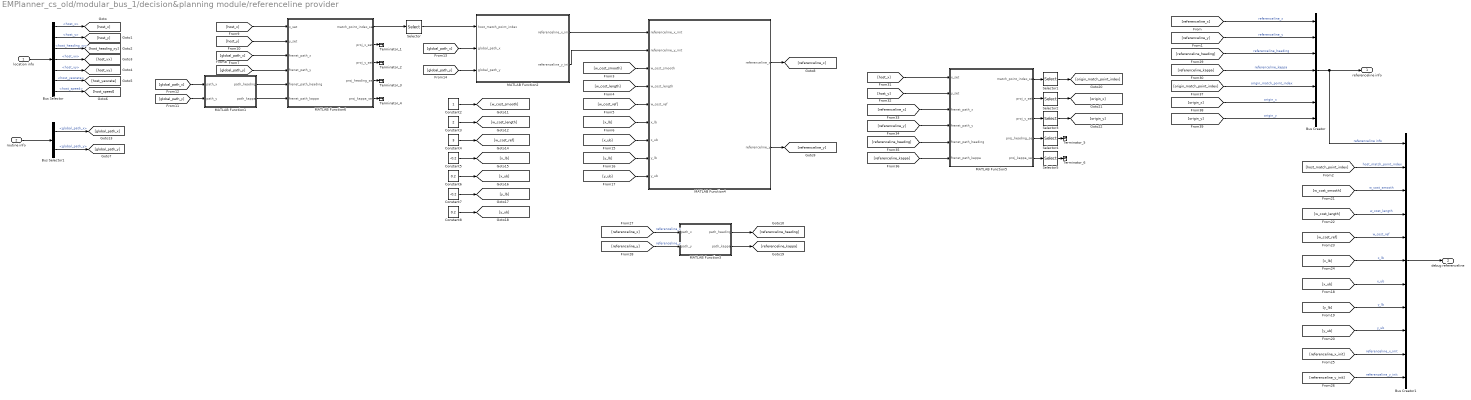
== system EMPlanner_cs_old/modular_bus_1/decision&planning module/referenceline provider ==
  location info : Inport
  routine info : Inport  Port=2
  Bus Creator : BusCreator  Inputs=7
  Bus Creator1 : BusCreator  Inputs=11
  Bus Selector : BusSelector  OutputSignals=host_x,host_y,host_heading_xy,host_vx,host_vy,host_yawrate,host_speed
  Bus Selector1 : BusSelector  OutputSignals=global_path_x,global_path_y
  Constant2 : Constant
  Constant3 : Constant  Value=2
  Constant4 : Constant  Value=3
  Constant5 : Constant  Value=-0.2
  Constant6 : Constant  Value=0.2
  Constant7 : Constant  Value=-0.2
  Constant8 : Constant  Value=0.2
  MATLAB Function1 : MATLAB Function  TreatAsAtomicUnit=on
  MATLAB Function2 : MATLAB Function  TreatAsAtomicUnit=on
  MATLAB Function3 : MATLAB Function  TreatAsAtomicUnit=on
  MATLAB Function4 : MATLAB Function  TreatAsAtomicUnit=on
  MATLAB Function5 : MATLAB Function  TreatAsAtomicUnit=on
  MATLAB Function6 : MATLAB Function  TreatAsAtomicUnit=on
  Selector{,1..5} (6 alike) : Selector  InputPortWidth=128  IndexOptions=Index vector (dialog)  Indices=1  OutputSizes=1
  Terminator_{1..6} (6 alike) : Terminator
  referenceline info : Outport
  debug referenceline : Outport  Port=2
  wires:
  Selector5/1 -> Terminator_6/1
  Selector4/1 -> Terminator_5/1
  MATLAB Function6/5(proj_kappa_set) -> Terminator_4/1
  MATLAB Function6/4(proj_heading_set) -> Terminator_3/1
  MATLAB Function6/3(proj_y_set) -> Terminator_2/1
  MATLAB Function6/2(proj_x_set) -> Terminator_1/1
  [origin_y] -> Bus Creator/7  "origin_y"
  [origin_x] -> Bus Creator/6  "origin_x"
  [origin_match_point_index] -> Bus Creator/5  "origin_match_point_index"
  Selector3/1 -> [origin_y]
  Selector2/1 -> [origin_x]
  Selector1/1 -> [origin_match_point_index]
  MATLAB Function5/5(proj_kappa_set) -> Selector5/1
  MATLAB Function5/4(proj_heading_set) -> Selector4/1
  MATLAB Function5/3(proj_y_set) -> Selector3/1
  MATLAB Function5/2(proj_x_set) -> Selector2/1
  MATLAB Function5/1(match_point_index_set) -> Selector1/1
  [referenceline_kappa] -> MATLAB Function5/6(frenet_path_kappa)
  [referenceline_heading] -> MATLAB Function5/5(frenet_path_heading)
  [referenceline_y] -> MATLAB Function5/4(frenet_path_y)
  [referenceline_x] -> MATLAB Function5/3(frenet_path_x)
  [host_y] -> MATLAB Function5/2(y_set)
  [host_x] -> MATLAB Function5/1(x_set)
  [referenceline_heading] -> Bus Creator/3  "referenceline_heading"
  [referenceline_kappa] -> Bus Creator/4  "referenceline_kappa"
  MATLAB Function3/2(path_kappa) -> [referenceline_kappa]
  MATLAB Function3/1(path_heading) -> [referenceline_heading]
  [referenceline_y] -> MATLAB Function3/2(path_y)  "referenceline_y"
  [referenceline_x] -> MATLAB Function3/1(path_x)  "referenceline_x"
  [referenceline_y_init] -> Bus Creator1/11  "referenceline_y_init"
  [referenceline_x_init] -> Bus Creator1/10  "referenceline_x_init"
  [y_ub] -> Bus Creator1/9  "y_ub"
  [host_match_point_index] -> Bus Creator1/2  "host_match_point_index"
  [y_lb] -> Bus Creator1/8  "y_lb"
  [w_cost_smooth] -> Bus Creator1/3  "w_cost_smooth"
  [x_ub] -> Bus Creator1/7  "x_ub"
  [w_cost_length] -> Bus Creator1/4  "w_cost_length"
  [x_lb] -> Bus Creator1/6  "x_lb"
  [w_cost_ref] -> Bus Creator1/5  "w_cost_ref"
  MATLAB Function2/2(referenceline_y_init) -> MATLAB Function4/2(referenceline_y_init)
  [y_ub] -> MATLAB Function4/9(y_ub)
  [y_lb] -> MATLAB Function4/8(y_lb)
  [x_ub] -> MATLAB Function4/7(x_ub)
  [x_lb] -> MATLAB Function4/6(x_lb)
  [w_cost_ref] -> MATLAB Function4/5(w_cost_ref)
  [w_cost_length] -> MATLAB Function4/4(w_cost_length)
  [w_cost_smooth] -> MATLAB Function4/3(w_cost_smooth)
  Constant4/1 -> [w_cost_ref]
  Constant5/1 -> [x_lb]
  Constant6/1 -> [x_ub]
  Constant7/1 -> [y_lb]
  Constant8/1 -> [y_ub]
  Constant3/1 -> [w_cost_length]
  Constant2/1 -> [w_cost_smooth]
  Bus Creator/1 -> referenceline info/1, Bus Creator1/1  "referenceline info"
  Bus Creator1/1 -> debug referenceline/1
  [referenceline_y] -> Bus Creator/2  "referenceline_y"
  [referenceline_x] -> Bus Creator/1  "referenceline_x"
  MATLAB Function4/2(referenceline_y) -> [referenceline_y]
  MATLAB Function4/1(referenceline_x) -> [referenceline_x]
  routine info/1 -> Bus Selector1/1
  Bus Selector1/1 -> [global_path_x]  "<global_path_x>"
  Bus Selector1/2 -> [global_path_y]  "<global_path_y>"
  location info/1 -> Bus Selector/1
  Bus Selector/6 -> [host_yawrate]  "<host_yawrate>"
  Bus Selector/7 -> [host_speed]  "<host_speed>"
  Bus Selector/4 -> [host_vx]  "<host_vx>"
  Bus Selector/3 -> [host_heading_xy]  "<host_heading_xy>"
  Bus Selector/2 -> [host_y]  "<host_y>"
  Bus Selector/1 -> [host_x]  "<host_x>"
  Bus Selector/5 -> [host_vy]  "<host_vy>"
  MATLAB Function2/1(referenceline_x_init) -> MATLAB Function4/1(referenceline_x_init)
  [global_path_y] -> MATLAB Function2/3(global_path_y)
  MATLAB Function6/1(match_point_index_set) -> Selector/1
  Selector/1 -> MATLAB Function2/1(host_match_point_index)
  [global_path_x] -> MATLAB Function1/1(path_x)
  [global_path_y] -> MATLAB Function1/2(path_y)
  [host_y] -> MATLAB Function6/2(y_set)
  [global_path_x] -> MATLAB Function6/3(frenet_path_x)
  [global_path_y] -> MATLAB Function6/4(frenet_path_y)
  MATLAB Function1/1(path_heading) -> MATLAB Function6/5(frenet_path_heading)
  MATLAB Function1/2(path_kappa) -> MATLAB Function6/6(frenet_path_kappa)
  [host_x] -> MATLAB Function6/1(x_set)
  [global_path_x] -> MATLAB Function2/2(global_path_x)

== system EMPlanner_cs_old/Box_1/SELF_Demux/compas converter/cart2compas ==
  Angle [deg] : Inport
  Constant : Constant  Value=90
  Constant1 : Constant  Value=360
  Gain : Gain  Gain=1/360
  Gain1 : Gain  Gain=360
  Gain2 : Gain  Gain=-1
  Rounding Function : Rounding
  Sum : Sum  Inputs=|-+
  Sum1 : Sum  Inputs=-+|
  Sum2 : Sum  Inputs=++|
  heading [deg] : Outport
  wires:
  Gain/1 -> Rounding Function/1
  Rounding Function/1 -> Gain1/1
  Gain1/1 -> Sum/1
  Angle [deg]/1 -> Sum1/2
  Sum/1 -> Gain2/1
  Sum1/1 -> Gain/1, Sum/2
  Constant/1 -> Sum1/1
  Gain2/1 -> Sum2/2
  Constant1/1 -> Sum2/1
  Sum2/1 -> heading [deg]/1

== system EMPlanner_cs_old/Box_10/SELF_Demux/compas converter/cart2compas ==
  Angle [deg] : Inport
  Constant : Constant  Value=90
  Constant1 : Constant  Value=360
  Gain : Gain  Gain=1/360
  Gain1 : Gain  Gain=360
  Gain2 : Gain  Gain=-1
  Rounding Function : Rounding
  Sum : Sum  Inputs=|-+
  Sum1 : Sum  Inputs=-+|
  Sum2 : Sum  Inputs=++|
  heading [deg] : Outport
  wires:
  Gain/1 -> Rounding Function/1
  Rounding Function/1 -> Gain1/1
  Gain1/1 -> Sum/1
  Angle [deg]/1 -> Sum1/2
  Sum/1 -> Gain2/1
  Sum1/1 -> Gain/1, Sum/2
  Constant/1 -> Sum1/1
  Gain2/1 -> Sum2/2
  Constant1/1 -> Sum2/1
  Sum2/1 -> heading [deg]/1

== system EMPlanner_cs_old/Box_2/SELF_Demux/compas converter/cart2compas ==
  Angle [deg] : Inport
  Constant : Constant  Value=90
  Constant1 : Constant  Value=360
  Gain : Gain  Gain=1/360
  Gain1 : Gain  Gain=360
  Gain2 : Gain  Gain=-1
  Rounding Function : Rounding
  Sum : Sum  Inputs=|-+
  Sum1 : Sum  Inputs=-+|
  Sum2 : Sum  Inputs=++|
  heading [deg] : Outport
  wires:
  Gain/1 -> Rounding Function/1
  Rounding Function/1 -> Gain1/1
  Gain1/1 -> Sum/1
  Angle [deg]/1 -> Sum1/2
  Sum/1 -> Gain2/1
  Sum1/1 -> Gain/1, Sum/2
  Constant/1 -> Sum1/1
  Gain2/1 -> Sum2/2
  Constant1/1 -> Sum2/1
  Sum2/1 -> heading [deg]/1

== system EMPlanner_cs_old/Box_3/SELF_Demux/compas converter/cart2compas ==
  Angle [deg] : Inport
  Constant : Constant  Value=90
  Constant1 : Constant  Value=360
  Gain : Gain  Gain=1/360
  Gain1 : Gain  Gain=360
  Gain2 : Gain  Gain=-1
  Rounding Function : Rounding
  Sum : Sum  Inputs=|-+
  Sum1 : Sum  Inputs=-+|
  Sum2 : Sum  Inputs=++|
  heading [deg] : Outport
  wires:
  Gain/1 -> Rounding Function/1
  Rounding Function/1 -> Gain1/1
  Gain1/1 -> Sum/1
  Angle [deg]/1 -> Sum1/2
  Sum/1 -> Gain2/1
  Sum1/1 -> Gain/1, Sum/2
  Constant/1 -> Sum1/1
  Gain2/1 -> Sum2/2
  Constant1/1 -> Sum2/1
  Sum2/1 -> heading [deg]/1

== system EMPlanner_cs_old/Box_4/SELF_Demux/compas converter/cart2compas ==
  Angle [deg] : Inport
  Constant : Constant  Value=90
  Constant1 : Constant  Value=360
  Gain : Gain  Gain=1/360
  Gain1 : Gain  Gain=360
  Gain2 : Gain  Gain=-1
  Rounding Function : Rounding
  Sum : Sum  Inputs=|-+
  Sum1 : Sum  Inputs=-+|
  Sum2 : Sum  Inputs=++|
  heading [deg] : Outport
  wires:
  Gain/1 -> Rounding Function/1
  Rounding Function/1 -> Gain1/1
  Gain1/1 -> Sum/1
  Angle [deg]/1 -> Sum1/2
  Sum/1 -> Gain2/1
  Sum1/1 -> Gain/1, Sum/2
  Constant/1 -> Sum1/1
  Gain2/1 -> Sum2/2
  Constant1/1 -> Sum2/1
  Sum2/1 -> heading [deg]/1

== system EMPlanner_cs_old/Box_5/SELF_Demux/compas converter/cart2compas ==
  Angle [deg] : Inport
  Constant : Constant  Value=90
  Constant1 : Constant  Value=360
  Gain : Gain  Gain=1/360
  Gain1 : Gain  Gain=360
  Gain2 : Gain  Gain=-1
  Rounding Function : Rounding
  Sum : Sum  Inputs=|-+
  Sum1 : Sum  Inputs=-+|
  Sum2 : Sum  Inputs=++|
  heading [deg] : Outport
  wires:
  Gain/1 -> Rounding Function/1
  Rounding Function/1 -> Gain1/1
  Gain1/1 -> Sum/1
  Angle [deg]/1 -> Sum1/2
  Sum/1 -> Gain2/1
  Sum1/1 -> Gain/1, Sum/2
  Constant/1 -> Sum1/1
  Gain2/1 -> Sum2/2
  Constant1/1 -> Sum2/1
  Sum2/1 -> heading [deg]/1

== system EMPlanner_cs_old/Box_6/SELF_Demux/compas converter/cart2compas ==
  Angle [deg] : Inport
  Constant : Constant  Value=90
  Constant1 : Constant  Value=360
  Gain : Gain  Gain=1/360
  Gain1 : Gain  Gain=360
  Gain2 : Gain  Gain=-1
  Rounding Function : Rounding
  Sum : Sum  Inputs=|-+
  Sum1 : Sum  Inputs=-+|
  Sum2 : Sum  Inputs=++|
  heading [deg] : Outport
  wires:
  Gain/1 -> Rounding Function/1
  Rounding Function/1 -> Gain1/1
  Gain1/1 -> Sum/1
  Angle [deg]/1 -> Sum1/2
  Sum/1 -> Gain2/1
  Sum1/1 -> Gain/1, Sum/2
  Constant/1 -> Sum1/1
  Gain2/1 -> Sum2/2
  Constant1/1 -> Sum2/1
  Sum2/1 -> heading [deg]/1

== system EMPlanner_cs_old/Box_7/SELF_Demux/compas converter/cart2compas ==
  Angle [deg] : Inport
  Constant : Constant  Value=90
  Constant1 : Constant  Value=360
  Gain : Gain  Gain=1/360
  Gain1 : Gain  Gain=360
  Gain2 : Gain  Gain=-1
  Rounding Function : Rounding
  Sum : Sum  Inputs=|-+
  Sum1 : Sum  Inputs=-+|
  Sum2 : Sum  Inputs=++|
  heading [deg] : Outport
  wires:
  Gain/1 -> Rounding Function/1
  Rounding Function/1 -> Gain1/1
  Gain1/1 -> Sum/1
  Angle [deg]/1 -> Sum1/2
  Sum/1 -> Gain2/1
  Sum1/1 -> Gain/1, Sum/2
  Constant/1 -> Sum1/1
  Gain2/1 -> Sum2/2
  Constant1/1 -> Sum2/1
  Sum2/1 -> heading [deg]/1

== system EMPlanner_cs_old/Box_8/SELF_Demux/compas converter/cart2compas ==
  Angle [deg] : Inport
  Constant : Constant  Value=90
  Constant1 : Constant  Value=360
  Gain : Gain  Gain=1/360
  Gain1 : Gain  Gain=360
  Gain2 : Gain  Gain=-1
  Rounding Function : Rounding
  Sum : Sum  Inputs=|-+
  Sum1 : Sum  Inputs=-+|
  Sum2 : Sum  Inputs=++|
  heading [deg] : Outport
  wires:
  Gain/1 -> Rounding Function/1
  Rounding Function/1 -> Gain1/1
  Gain1/1 -> Sum/1
  Angle [deg]/1 -> Sum1/2
  Sum/1 -> Gain2/1
  Sum1/1 -> Gain/1, Sum/2
  Constant/1 -> Sum1/1
  Gain2/1 -> Sum2/2
  Constant1/1 -> Sum2/1
  Sum2/1 -> heading [deg]/1

== system EMPlanner_cs_old/Box_9/SELF_Demux/compas converter/cart2compas ==
  Angle [deg] : Inport
  Constant : Constant  Value=90
  Constant1 : Constant  Value=360
  Gain : Gain  Gain=1/360
  Gain1 : Gain  Gain=360
  Gain2 : Gain  Gain=-1
  Rounding Function : Rounding
  Sum : Sum  Inputs=|-+
  Sum1 : Sum  Inputs=-+|
  Sum2 : Sum  Inputs=++|
  heading [deg] : Outport
  wires:
  Gain/1 -> Rounding Function/1
  Rounding Function/1 -> Gain1/1
  Gain1/1 -> Sum/1
  Angle [deg]/1 -> Sum1/2
  Sum/1 -> Gain2/1
  Sum1/1 -> Gain/1, Sum/2
  Constant/1 -> Sum1/1
  Gain2/1 -> Sum2/2
  Constant1/1 -> Sum2/1
  Sum2/1 -> heading [deg]/1
